simulink model "planta_inicial_tune"  (R2025b)
settings: Solver=VariableStepAuto  StartTime=0.0  StopTime=15  RelTol=1e-3
model workspace (MAT data in the model file):
  w = 0.5
values from neighbouring files (symbols this model uses):
  C1 = 1.2801    [Data_ControleLateral_atual.m]
  C2 = 23.99    [Data_ControleLateral_atual.m]
  C3 = 0.52    [Data_ControleLateral_atual.m]
undefined symbols (not defined in the file or in its folder): EV, GND, MTR, WHL
libraries: slpidlib x3, autolibutils x2, autolibmappedmotor x2, vehdynlibviscommon x1, autolibshared x1
settings Model: PacingRate=0.500000  Creator=Guilherme Porto  LastModifiedBy=Guilherme Porto

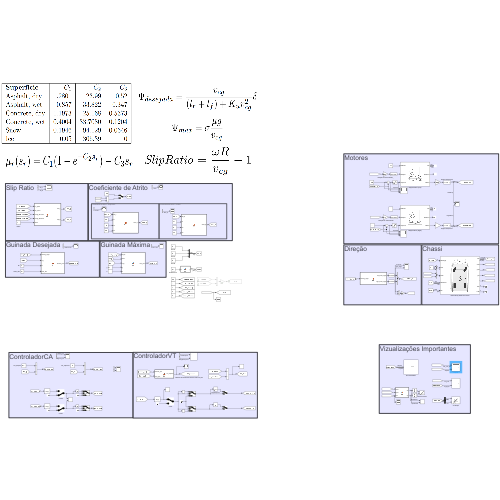
[thumbnail: Simulink's stored preview of the top-level diagram]
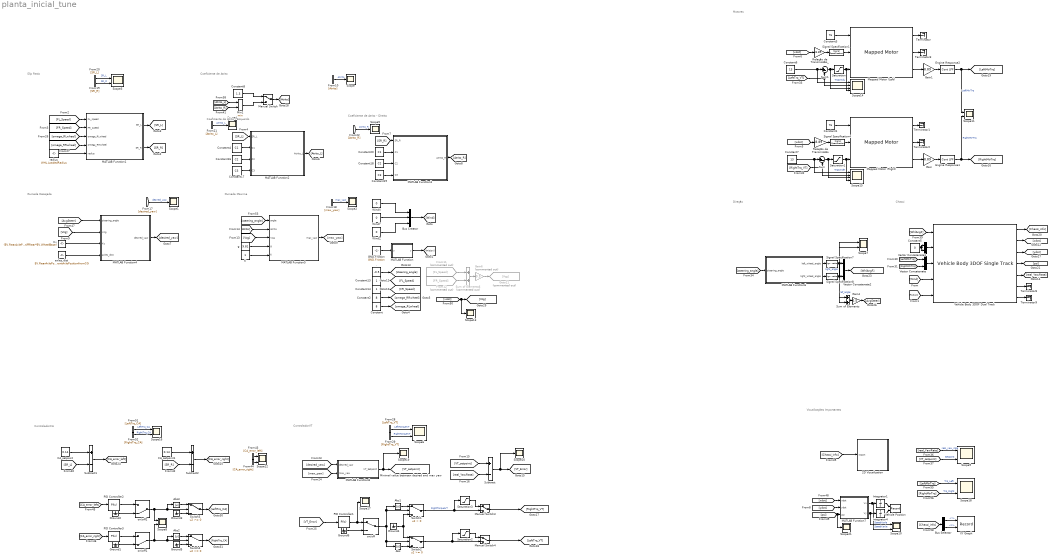
== system planta_inicial_tune ==
  note: Motores
  note: Direção
  note: Guinada Máxima
  note: Guinada Desejada
  note: Coeficiente de Atrito
  note: Coeficiente de Atrito - Esquerdo
  note: Slip Ratio
  note: Coeficiente de Atrito - Direito
  note: ControladorVT
  note: ControladorCA
  note: Chassi
  note: Vizualizações Importantes
  . : Constant  Value=-0.5
  2D Visualization : Subsystem
      mask Display: image("visualization.JPG");
  Abs{,1..3} (4 alike) : Abs  SaturateOnIntegerOverflow=off
  Bus Creator : BusCreator  Inputs=3
  Bus Selector : BusSelector  OutputSignals=InertFrm.Cg.Disp.Y,InertFrm.Cg.Disp.X
  CA_setpoint : Constant  Value=0.14
  CA_setpoint1 : Constant  Value=0.14
  Constant : Constant  Value=8
  Constant1 : Constant  Value=76
  Constant13 : Constant
  Constant14 : Constant
  Constant16 : Constant  Value=C2
  Constant17 : Constant  Value=C3
  Constant18 : Constant  Value=C2
  Constant19 : Constant  Value=C3
  Constant2 : Constant  Value=8
  Constant20 : Constant  Value=C1
  Constant3 : Constant  Value=76
  Constant4 : Constant  Value=C1
  Constant5 : Constant  Value=0
  Constant6 : Constant  Value=13
  Constant7 : Constant  Value=13
  Constant8 : Constant  Value=1.3
  Engine Response1 : autolibutils/Cont LPF  wc=40*2*pi  AbsoluteTolerance=auto  aMode=2
  Engine Response2 : autolibutils/Cont LPF  wc=40*2*pi  AbsoluteTolerance=auto  aMode=2
  From11 : From  Commented=on  GotoTag=FL_Speed
  From12 : From  Commented=on  GotoTag=FR_Speed
  GND.Friction : Constant  Value=GND.Friction
  Gain : Gain  Gain=8.89
  Gain1 : Gain  Gain=8.89
  Gain4 : Gain  Gain=0.5
  Gain6 : Gain  Commented=on  Gain=0.5
  Goto11 : Goto  Commented=on  GotoTag=Vcg
  Ground{1..6} (6 alike) : Ground
  Integrator1 : Integrator
  Integrator4 : Integrator
  Ku : Constant  Value=(EV.RearAxlePositionfromCG*EV.Mass)/(EV.CornerStiffFront *EV.WheelBase)-(EV.FrontAxlePositionfromCG*EV.Mass)/(EV.CornerStiffRear*EV.WheelBase)
  MATLAB Function : MATLAB Function  TreatAsAtomicUnit=on
  MATLAB Function1 : MATLAB Function  TreatAsAtomicUnit=on
  MATLAB Function2 : MATLAB Function  TreatAsAtomicUnit=on
  MATLAB Function3 : MATLAB Function  TreatAsAtomicUnit=on
  MATLAB Function4 : MATLAB Function  TreatAsAtomicUnit=on
  MATLAB Function5 : MATLAB Function  TreatAsAtomicUnit=on
  MATLAB Function6 : MATLAB Function  TreatAsAtomicUnit=on
  MATLAB Function7 : MATLAB Function  TreatAsAtomicUnit=on
  MATLAB Function8 : MATLAB Function  TreatAsAtomicUnit=on
  Manual Switch : ManualSwitch
  Manual Switch3 : ManualSwitch
  Manual Switch4 : ManualSwitch
  Mapped Motor (Left) : autolibmappedmotor/Mapped Motor  w_Tmax_bp_ext=[-800;-750;-375;0;375;750;800]  Tmax_w_V_ext=[0 0 0;0.07 0.07 0.07;0.08 0.08 0.08;0.09 0.09 0.09;0.08 0.08 0.08;0.07 0.07 0.07;0 0 0]  w_Tmin_bp_ext=[-800;-750;-375;0;375;750;800]  Tmin_w_V_ext=[0 0 0;-0.07 -0.07 -0.07;-0.08 -0.08 -0.08;-0.09 -0.09 -0.09;-0.08 -0.08 -0.08;-0.07 -0.07 -0.07;0 0 0]  port_config=Speed  param_by=Tabulated torque-speed envelope  w_t=MTR.Speed  T_t=MTR.Torque*MTR.Overpower  torque_max=.1  power_max=30  SpreadsheetTqLimitsFileName=MotorCalibrationImportData.xlsx  Tmax_w_V=[0.09 0.09 0.09;0.08 0.08 0.08;0.07 0.07 0.07;0 0 0]  w_Tmax_bp=[ 0 375 750 800 ]  V_Tmax_bp=[500 750 900]  Tmin_w_V=[-0.09 -0.09 -0.09;-0.08 -0.08 -0.08;-0.07 -0.07 -0.07;0 0 0]  w_Tmin_bp=[ 0 375 750 800 ]  V_Tmin_bp=[500 750 900]  Tc=0.05  param_loss=Single efficiency measurement  SpreadsheetLossFileName=MotorCalibrationImportData.xlsx  SpreadsheetEffFileName=MotorCalibrationImportData.xlsx  eff=100  w_eff=375  T_eff=0.08  Piron=0  Pbase=0  w_eff_bp=[-800 -400 0 400 800]  T_eff_bp=[0 0.03 0.06 0.09]  Temp_eff_bp=[233.15 293.15 373.15]  V_eff_bp=[500 700 900]  losses_table=[1.49 1.67 2.21 3.10; 0.42 0.69 1.14 2.03; 0.06 0.24 0.78 1.68; 0.42 0.69 1.14 2.03; 1.49 1.67 2.21 3.10]  losses_table_3d=cat(3,[1.49 1.67 2.21 3.10; 0.42 0.69 1.14 2.03; 0.06 0.24 0.78 1.68; 0.42 0.69 1.14 2.03; 1.49 1.67 2.21 3.10],[1.49 1.67 2.21 3.10; 0.42 0.69 1.14 2.03; 0.06 0.24 0.78 1.68; 0.42 0.69 1.14 2.03; 1.49 1.67 2.21 3.10],[1.49 1.67 2.21 3.10; 0.42 0.69 1.14 2.03; 0.06 0.24 0.78 1.68; 0.42 0.69 1.14 2.03; 1.49 1.67 2.21 3.10])  losses_table_4d=cat(4,cat(3,[1.5645 0.441 0.063 0.441 1.5645;1.7535 0.7245 0.252 0.7245 1.7535;2.3205 1.197 0.819 1.197 2.3205;3.255 2.1315 1.764 2.1315 3.255],[1.5645 0.441 0.063 0.441 1.5645;1.7535 0.7245 0.252 0.7245 1.7535;2.3205 1.197 0.819 1.197 2.3205;3.255 2.1315 1.764 2.1315 3.255],[1.5645 0.441 0.063 0.441 1.5645;1.7535 0.7245 0.252 0.7245 1.7535;2.3205 1.197 0.819 1.197 2.3205;3.255 2.1315 1.764 2.1315 3.255]),cat(3,[1.49 0.42 0.06 0.42 1.49;1.67 0.69 0.24 0.69 1.67;2.21 1.14 0.78 1.14 2.21;3.1 2.03 1.68 2.03 3.1],[1.49 0.42 0.06 0.42 1.49;1.67 0.69 0.24 0.69 1.67;2.21 1.14 0.78 1.14 2.21;3.1 2.03 1.68 2.03 3.1],[1.49 0.42 0.06 0.42 1.49;1.67 0.69 0.24 0.69 1.67;2.21 1.14 0.78 1.14 2.21;3.1 2.03 1.68 2.03 3.1]),cat(3,[1.5347 0.4326 0.0618 0.4326 1.5347;1.7201 0.7107 0.2472 0.7107 1.7201;2.2763 1.1742 0.8034 1.1742 2.2763;3.193 2.0909 1.7304 2.0909 3.193],[1.5347 0.4326 0.0618 0.4326 1.5347;1.7201 0.7107 0.2472 0.7107 1.7201;2.2763 1.1742 0.8034 1.1742 2.2763;3.193 2.0909 1.7304 2.0909 3.193],[1.5347 0.4326 0.0618 0.4326 1.5347;1.7201 0.7107 0.2472 0.7107 1.7201;2.2763 1.1742 0.8034 1.1742 2.2763;3.193 2.0909 1.7304 2.0909 3.193]))  efficiency_table=[95 95 95 95; 95 95 95 95; 95 95 95 95; 95 95 95 95; 95 95 95 95]  efficiency_table_3d=cat(3,[95 95 95 95; 95 95 95 95; 95 95 95 95; 95 95 95 95; 95 95 95 95],[95 95 95 95; 95 95 95 95; 95 95 95 95; 95 95 95 95; 95 95 95 95],[95 95 95 95; 95 95 95 95; 95 95 95 95; 95 95 95 95; 95 95 95 95])  efficiency_table_4d=cat(4,cat(3,90*ones(5,4)',90*ones(5,4)',90*ones(5,4)'),cat(3,95*ones(5,4)',95*ones(5,4)',95*ones(5,4)'),cat(3,92*ones(5,4)',92*ones(5,4)',92*ones(5,4)'))  J=5e-6  b=1e-5  omega_o=0  T_t_extended=[0 0.07 0.08 0.09 0.08 0.07 0]  w_t_extended=[-800 -750 -375 0 375 750 800]  KLossIron=0  KLossCopper=0  x_w_eff_vec=[-8000 -4000 0 4000 8000]  x_T_eff_vec=[-0.09 -0.06 -0.03 0 0.03 0.06 0.09]  x_tmp_eff_vec=[-0.09 -0.06 -0.03 0 0.03 0.06 0.09]  x_V_eff_vec=[500 700 900]  x_losses_mat=[3.1 2.21 1.67 1.49 1.67 2.21 3.1;2.03 1.14 0.69 0.42 0.69 1.14 2.03;1.68 0.78 0.24 0.06 0.24 0.78 1.68;2.03 1.14 0.69 0.42 0.69 1.14 2.03;3.1 2.21 1.67 1.49 1.67 2.21 3.1]  x_losses_mat_3d=[37.8947368421052 25.2631578947368 12.6315789473684 0 12 24 36;18.9473684210526 12.6315789473684 6.3157894736842 0 5.99999999999999 12 18;0 0 0 0 0 0 0;18 12 5.99999999999999 0 6.3157894736842 12.6315789473684 18.9473684210526;36 24 12 0 12.6315789473684 25.2631578947368 37.8947368421052]  x_losses_mat_4d="reshape([80;53.33;26.67;0;24;48;72;40;26.67;13.33;0;12;24;36;0;0;0;0;0;0;0;36;24;12;0;13.33;26.67;40;72;48;24;0;26.67;53.33;80;80;53.33;26.67;0;24;48;72;40;26.67;13.33;0;12;24;36;0;0;0;0;0;0;0;36;24;12;0;13.33;26.67;40;72;48;24;0;26.67;53.33;80;80;53.33;26.67;0;24;48;72;40;26.67;13.33;0;12;24;36;0;0;0;0;0;0;0;36;24;12;0;13.33;26.67;40;72;48;24;0;26.67;53.33;80;37.89;25.26;12.63;0;12;24;36;18.95;12.63;6.32;0;6;12;18;0;0;0;0;0;0;0;18;12;6;0;6.32;12.63;18.95;36;24;12;0;12.63;25.26;37.89;37.89;25.26;12.63;0;12;24;36;18.95;12.63;6.32;0;6;12;18;0;0;0;0;0;0;0;18;12;6;0;6.32;12.63;18.95;36;24;12;0;12.63;25.26;37.89;37.89;25.26;12.63;0;12;24;36;18.95;12.63;6.32;0;6;12;18;0;0;0;0;0;0;0;18;12;6;0;6.32;12.63;18.95;36;24;12;0;12.63;25.26;37.89;62.61;41.74;20.87;0;19.2;38.4;57.6;31.3;20.87;10.43;0;9.6;19.2;28.8;0;0;0;0;0;0;0;28.8;19.2;9.6;0;10.43;20.87;31.3;57.6;38.4;19.2;0;20.87;41.74;62.61;62.61;41.74;20.87;0;19.2;38.4;57.6;31.3;20.87;10.43;0;9.6;19.2;28.8;0;0;0;0;0;0;0;28.8;19.2;9.6;0;10.43;20.87;31.3;57.6;38.4;19.2;0;20.87;41.74;62.61;62.61;41.74;20.87;0;19.2;38.4;57.6;31.3;20.87;10.43;0;9.6;19.2;28.8;0;0;0;0;0;0;0;28.8;19.2;9.6;0;10.43;20.87;31.3;57.6;38.4;19.2;0;20.87;41.74;62.61], [7  5  3  3])"  CalLossMapData={}  CalLossWithTempMapData={}  aMode=1  RefBlkName='autolibmappedmotor/Mapped Motor'
      settings: LibrarySourceBlock=autolibemachines/Mapped Motor
  Mapped Motor (Right) : autolibmappedmotor/Mapped Motor  w_Tmax_bp_ext=[-800;-750;-375;0;375;750;800]  Tmax_w_V_ext=[0 0 0;0.07 0.07 0.07;0.08 0.08 0.08;0.09 0.09 0.09;0.08 0.08 0.08;0.07 0.07 0.07;0 0 0]  w_Tmin_bp_ext=[-800;-750;-375;0;375;750;800]  Tmin_w_V_ext=[0 0 0;-0.07 -0.07 -0.07;-0.08 -0.08 -0.08;-0.09 -0.09 -0.09;-0.08 -0.08 -0.08;-0.07 -0.07 -0.07;0 0 0]  port_config=Speed  param_by=Tabulated torque-speed envelope  w_t=MTR.Speed  T_t=MTR.Torque*MTR.Overpower  torque_max=.1  power_max=30  SpreadsheetTqLimitsFileName=MotorCalibrationImportData.xlsx  Tmax_w_V=[0.09 0.09 0.09;0.08 0.08 0.08;0.07 0.07 0.07;0 0 0]  w_Tmax_bp=[ 0 375 750 800 ]  V_Tmax_bp=[500 750 900]  Tmin_w_V=[-0.09 -0.09 -0.09;-0.08 -0.08 -0.08;-0.07 -0.07 -0.07;0 0 0]  w_Tmin_bp=[ 0 375 750 800 ]  V_Tmin_bp=[500 750 900]  Tc=0.05  param_loss=Single efficiency measurement  SpreadsheetLossFileName=MotorCalibrationImportData.xlsx  SpreadsheetEffFileName=MotorCalibrationImportData.xlsx  eff=100  w_eff=375  T_eff=0.08  Piron=0  Pbase=0  w_eff_bp=[-800 -400 0 400 800]  T_eff_bp=[0 0.03 0.06 0.09]  Temp_eff_bp=[233.15 293.15 373.15]  V_eff_bp=[500 700 900]  losses_table=[1.49 1.67 2.21 3.10; 0.42 0.69 1.14 2.03; 0.06 0.24 0.78 1.68; 0.42 0.69 1.14 2.03; 1.49 1.67 2.21 3.10]  losses_table_3d=cat(3,[1.49 1.67 2.21 3.10; 0.42 0.69 1.14 2.03; 0.06 0.24 0.78 1.68; 0.42 0.69 1.14 2.03; 1.49 1.67 2.21 3.10],[1.49 1.67 2.21 3.10; 0.42 0.69 1.14 2.03; 0.06 0.24 0.78 1.68; 0.42 0.69 1.14 2.03; 1.49 1.67 2.21 3.10],[1.49 1.67 2.21 3.10; 0.42 0.69 1.14 2.03; 0.06 0.24 0.78 1.68; 0.42 0.69 1.14 2.03; 1.49 1.67 2.21 3.10])  losses_table_4d=cat(4,cat(3,[1.5645 0.441 0.063 0.441 1.5645;1.7535 0.7245 0.252 0.7245 1.7535;2.3205 1.197 0.819 1.197 2.3205;3.255 2.1315 1.764 2.1315 3.255],[1.5645 0.441 0.063 0.441 1.5645;1.7535 0.7245 0.252 0.7245 1.7535;2.3205 1.197 0.819 1.197 2.3205;3.255 2.1315 1.764 2.1315 3.255],[1.5645 0.441 0.063 0.441 1.5645;1.7535 0.7245 0.252 0.7245 1.7535;2.3205 1.197 0.819 1.197 2.3205;3.255 2.1315 1.764 2.1315 3.255]),cat(3,[1.49 0.42 0.06 0.42 1.49;1.67 0.69 0.24 0.69 1.67;2.21 1.14 0.78 1.14 2.21;3.1 2.03 1.68 2.03 3.1],[1.49 0.42 0.06 0.42 1.49;1.67 0.69 0.24 0.69 1.67;2.21 1.14 0.78 1.14 2.21;3.1 2.03 1.68 2.03 3.1],[1.49 0.42 0.06 0.42 1.49;1.67 0.69 0.24 0.69 1.67;2.21 1.14 0.78 1.14 2.21;3.1 2.03 1.68 2.03 3.1]),cat(3,[1.5347 0.4326 0.0618 0.4326 1.5347;1.7201 0.7107 0.2472 0.7107 1.7201;2.2763 1.1742 0.8034 1.1742 2.2763;3.193 2.0909 1.7304 2.0909 3.193],[1.5347 0.4326 0.0618 0.4326 1.5347;1.7201 0.7107 0.2472 0.7107 1.7201;2.2763 1.1742 0.8034 1.1742 2.2763;3.193 2.0909 1.7304 2.0909 3.193],[1.5347 0.4326 0.0618 0.4326 1.5347;1.7201 0.7107 0.2472 0.7107 1.7201;2.2763 1.1742 0.8034 1.1742 2.2763;3.193 2.0909 1.7304 2.0909 3.193]))  efficiency_table=[95 95 95 95; 95 95 95 95; 95 95 95 95; 95 95 95 95; 95 95 95 95]  efficiency_table_3d=cat(3,[95 95 95 95; 95 95 95 95; 95 95 95 95; 95 95 95 95; 95 95 95 95],[95 95 95 95; 95 95 95 95; 95 95 95 95; 95 95 95 95; 95 95 95 95],[95 95 95 95; 95 95 95 95; 95 95 95 95; 95 95 95 95; 95 95 95 95])  efficiency_table_4d=cat(4,cat(3,90*ones(5,4)',90*ones(5,4)',90*ones(5,4)'),cat(3,95*ones(5,4)',95*ones(5,4)',95*ones(5,4)'),cat(3,92*ones(5,4)',92*ones(5,4)',92*ones(5,4)'))  J=5e-6  b=1e-5  omega_o=0  T_t_extended=[0 0.07 0.08 0.09 0.08 0.07 0]  w_t_extended=[-800 -750 -375 0 375 750 800]  KLossIron=0  KLossCopper=0  x_w_eff_vec=[-8000 -4000 0 4000 8000]  x_T_eff_vec=[-0.09 -0.06 -0.03 0 0.03 0.06 0.09]  x_tmp_eff_vec=[-0.09 -0.06 -0.03 0 0.03 0.06 0.09]  x_V_eff_vec=[500 700 900]  x_losses_mat=[3.1 2.21 1.67 1.49 1.67 2.21 3.1;2.03 1.14 0.69 0.42 0.69 1.14 2.03;1.68 0.78 0.24 0.06 0.24 0.78 1.68;2.03 1.14 0.69 0.42 0.69 1.14 2.03;3.1 2.21 1.67 1.49 1.67 2.21 3.1]  x_losses_mat_3d=[37.8947368421052 25.2631578947368 12.6315789473684 0 12 24 36;18.9473684210526 12.6315789473684 6.3157894736842 0 5.99999999999999 12 18;0 0 0 0 0 0 0;18 12 5.99999999999999 0 6.3157894736842 12.6315789473684 18.9473684210526;36 24 12 0 12.6315789473684 25.2631578947368 37.8947368421052]  x_losses_mat_4d="reshape([80;53.33;26.67;0;24;48;72;40;26.67;13.33;0;12;24;36;0;0;0;0;0;0;0;36;24;12;0;13.33;26.67;40;72;48;24;0;26.67;53.33;80;80;53.33;26.67;0;24;48;72;40;26.67;13.33;0;12;24;36;0;0;0;0;0;0;0;36;24;12;0;13.33;26.67;40;72;48;24;0;26.67;53.33;80;80;53.33;26.67;0;24;48;72;40;26.67;13.33;0;12;24;36;0;0;0;0;0;0;0;36;24;12;0;13.33;26.67;40;72;48;24;0;26.67;53.33;80;37.89;25.26;12.63;0;12;24;36;18.95;12.63;6.32;0;6;12;18;0;0;0;0;0;0;0;18;12;6;0;6.32;12.63;18.95;36;24;12;0;12.63;25.26;37.89;37.89;25.26;12.63;0;12;24;36;18.95;12.63;6.32;0;6;12;18;0;0;0;0;0;0;0;18;12;6;0;6.32;12.63;18.95;36;24;12;0;12.63;25.26;37.89;37.89;25.26;12.63;0;12;24;36;18.95;12.63;6.32;0;6;12;18;0;0;0;0;0;0;0;18;12;6;0;6.32;12.63;18.95;36;24;12;0;12.63;25.26;37.89;62.61;41.74;20.87;0;19.2;38.4;57.6;31.3;20.87;10.43;0;9.6;19.2;28.8;0;0;0;0;0;0;0;28.8;19.2;9.6;0;10.43;20.87;31.3;57.6;38.4;19.2;0;20.87;41.74;62.61;62.61;41.74;20.87;0;19.2;38.4;57.6;31.3;20.87;10.43;0;9.6;19.2;28.8;0;0;0;0;0;0;0;28.8;19.2;9.6;0;10.43;20.87;31.3;57.6;38.4;19.2;0;20.87;41.74;62.61;62.61;41.74;20.87;0;19.2;38.4;57.6;31.3;20.87;10.43;0;9.6;19.2;28.8;0;0;0;0;0;0;0;28.8;19.2;9.6;0;10.43;20.87;31.3;57.6;38.4;19.2;0;20.87;41.74;62.61], [7  5  3  3])"  CalLossMapData={'BaseCageProjectFileName','';'BaseMbcProjectFileName','';'TaskName','Calibrate Motor Loss Map';'ChildTasks',{{'DataName','';'TaskName','Import Loss Data'},{'TaskName','Generate Response Models'},{'TaskName','Generate Calibration'},{'TaskName','Update Block Parameters'}}}  CalLossWithTempMapData={}  aMode=1  RefBlkName='autolibmappedmotor/Mapped Motor'
      settings: LibrarySourceBlock=autolibemachines/Mapped Motor
  Min1 : MinMax  Inputs=2
  PID Controller1 : slpidlib/PID Controller  Controller=PI  Form=Parallel  TimeDomain=Continuous-time  UseExternalTs=off  SampleTime=-1  IntegratorMethod=Forward Euler  FilterMethod=Forward Euler  ControllerParametersSource=internal  P=1188  I=86  UseKiTs=off  D=-1.04450033164761  UseExternalDerivativeSource=off  N=21.9051072982779  UseFilter=on  TunerSelectOption=Transfer Function Based (PID Tuner App)  InitialConditionSource=internal  InitialConditionForIntegrator=0  InitialConditionForFilter=0  DifferentiatorICPrevScaledInput=0  ExternalReset=none  TrackingMode=off  Kt=1  LimitOutput=off  SatLimitsSource=internal  UpperSaturationLimit=inf  LowerSaturationLimit=-inf  LinearizeAsGain=on  AntiWindupMode=none  Kb=1  LimitIntegrator=off  UpperIntegratorSaturationLimit=inf  LowerIntegratorSaturationLimit=-inf  POutMin=[]  POutMax=[]  IOutMin=[]  IOutMax=[]  DOutMin=[]  DOutMax=[]  NOutMin=[]  NOutMax=[]  SumOutMin=[]  SumOutMax=[]  SaturationOutMin=[]  SaturationOutMax=[]  PParamMin=[]  PParamMax=[]  IParamMin=[]  IParamMax=[]  DParamMin=[]  DParamMax=[]  NParamMin=[]  NParamMax=[]  KbParamMin=[]  KbParamMax=[]  KtParamMin=[]  KtParamMax=[]  KbOutMin=[]  KbOutMax=[]  KtOutMin=[]  KtOutMax=[]  IntegratorOutMin=[]  IntegratorOutMax=[]  FilterOutMin=[]  FilterOutMax=[]  SumI1OutMin=[]  SumI1OutMax=[]  SumI2OutMin=[]  SumI2OutMax=[]  SumI3OutMin=[]  SumI3OutMax=[]  SumI4OutMin=[]  SumI4OutMax=[]  SumDOutMin=[]  SumDOutMax=[]  DifferentiatorOutMin=[]  DifferentiatorOutMax=[]  FilterDiffOutCoefMin=[]  FilterDiffOutCoefMax=[]  ReciprocalOutMin=[]  ReciprocalOutMax=[]  SumDenOutMin=[]  SumDenOutMax=[]  SumNumOutMin=[]  SumNumOutMax=[]  DivideOutMin=[]  DivideOutMax=[]  UdiffTsProdOutMin=[]  UdiffTsProdOutMax=[]  NTsProdOutMin=[]  NTsProdOutMax=[]  UintegralTsProdOutMin=[]  UintegralTsProdOutMax=[]  UngainTsProdOutMin=[]  UngainTsProdOutMax=[]  ClampingZeroOutDataTypeStr=Inherit: Inherit via back propagation  ClampingZeroOutMin=[]  ClampingZeroOutMax=[]  FilterDenConstantOutDataTypeStr=Inherit: Inherit via back propagation  FilterDenConstantOutMin=[]  FilterDenConstantOutMax=[]  PCopyOutDataTypeStr=Inherit: Inherit via back propagation  PCopyOutMin=[]  PCopyOutMax=[]  NCopyOutDataTypeStr=Inherit: Inherit via back propagation  NCopyOutMin=[]  NCopyOutMax=[]  IntegratorContinuousStateAttributes=''  IntegratorStateMustResolveToSignalObject=off  IntegratorRTWStateStorageClass=Auto  FilterContinuousStateAttributes=''  FilterStateMustResolveToSignalObject=off  FilterRTWStateStorageClass=Auto  ParallelPVariant=InternalParameters  IdealPVariant=Disabled  IVariant=InternalParameters  DVariant=Disabled  IntegratorVariant=Continuous  SatVariant=Disabled  AWVariant=Passthrough  PCopyVariant=Disabled  TRVariant=Disabled  FdbkBlocksVariant=Forward  IdealPFdbkVariant=Disabled  SatFdbkVariant=Disabled  DerivativeFilterVariant=Disabled  NVariant=Disabled  NCopyVariant=Disabled_SignalSpec  FilterICVariant=Disabled  IntegratorICVariant=InternalICs  ExternalResetVariant=Disabled  TRSumVariant=Passthrough  SumFdbkVariant=Disabled  SumVariant=Sum_PI  TsampFilterVariant=InternalTs  TsampNgainVariant=Passthrough  TsampIntegralVariant=Disabled_SignalSpec  ExternalSaturationOutDataTypeStr=Inherit: Same as second input  DerivativeSourceVariant=Disabled  PreIntVariant=InternalPreInt
  PID Controller2 : slpidlib/PID Controller  Controller=PI  Form=Parallel  TimeDomain=Continuous-time  UseExternalTs=off  SampleTime=-1  IntegratorMethod=Forward Euler  FilterMethod=Forward Euler  ControllerParametersSource=internal  P=1000  I=100  UseKiTs=off  D=-1.04450033164761  UseExternalDerivativeSource=off  N=21.9051072982779  UseFilter=on  TunerSelectOption=Transfer Function Based (PID Tuner App)  InitialConditionSource=internal  InitialConditionForIntegrator=0  InitialConditionForFilter=0  DifferentiatorICPrevScaledInput=0  ExternalReset=none  TrackingMode=off  Kt=1  LimitOutput=off  SatLimitsSource=internal  UpperSaturationLimit=inf  LowerSaturationLimit=-inf  LinearizeAsGain=on  AntiWindupMode=none  Kb=1  LimitIntegrator=off  UpperIntegratorSaturationLimit=inf  LowerIntegratorSaturationLimit=-inf  POutMin=[]  POutMax=[]  IOutMin=[]  IOutMax=[]  DOutMin=[]  DOutMax=[]  NOutMin=[]  NOutMax=[]  SumOutMin=[]  SumOutMax=[]  SaturationOutMin=[]  SaturationOutMax=[]  PParamMin=[]  PParamMax=[]  IParamMin=[]  IParamMax=[]  DParamMin=[]  DParamMax=[]  NParamMin=[]  NParamMax=[]  KbParamMin=[]  KbParamMax=[]  KtParamMin=[]  KtParamMax=[]  KbOutMin=[]  KbOutMax=[]  KtOutMin=[]  KtOutMax=[]  IntegratorOutMin=[]  IntegratorOutMax=[]  FilterOutMin=[]  FilterOutMax=[]  SumI1OutMin=[]  SumI1OutMax=[]  SumI2OutMin=[]  SumI2OutMax=[]  SumI3OutMin=[]  SumI3OutMax=[]  SumI4OutMin=[]  SumI4OutMax=[]  SumDOutMin=[]  SumDOutMax=[]  DifferentiatorOutMin=[]  DifferentiatorOutMax=[]  FilterDiffOutCoefMin=[]  FilterDiffOutCoefMax=[]  ReciprocalOutMin=[]  ReciprocalOutMax=[]  SumDenOutMin=[]  SumDenOutMax=[]  SumNumOutMin=[]  SumNumOutMax=[]  DivideOutMin=[]  DivideOutMax=[]  UdiffTsProdOutMin=[]  UdiffTsProdOutMax=[]  NTsProdOutMin=[]  NTsProdOutMax=[]  UintegralTsProdOutMin=[]  UintegralTsProdOutMax=[]  UngainTsProdOutMin=[]  UngainTsProdOutMax=[]  ClampingZeroOutDataTypeStr=Inherit: Inherit via back propagation  ClampingZeroOutMin=[]  ClampingZeroOutMax=[]  FilterDenConstantOutDataTypeStr=Inherit: Inherit via back propagation  FilterDenConstantOutMin=[]  FilterDenConstantOutMax=[]  PCopyOutDataTypeStr=Inherit: Inherit via back propagation  PCopyOutMin=[]  PCopyOutMax=[]  NCopyOutDataTypeStr=Inherit: Inherit via back propagation  NCopyOutMin=[]  NCopyOutMax=[]  IntegratorContinuousStateAttributes=''  IntegratorStateMustResolveToSignalObject=off  IntegratorRTWStateStorageClass=Auto  FilterContinuousStateAttributes=''  FilterStateMustResolveToSignalObject=off  FilterRTWStateStorageClass=Auto  ParallelPVariant=InternalParameters  IdealPVariant=Disabled  IVariant=InternalParameters  DVariant=Disabled  IntegratorVariant=Continuous  SatVariant=Disabled  AWVariant=Passthrough  PCopyVariant=Disabled  TRVariant=Disabled  FdbkBlocksVariant=Forward  IdealPFdbkVariant=Disabled  SatFdbkVariant=Disabled  DerivativeFilterVariant=Disabled  NVariant=Disabled  NCopyVariant=Disabled_SignalSpec  FilterICVariant=Disabled  IntegratorICVariant=InternalICs  ExternalResetVariant=Disabled  TRSumVariant=Passthrough  SumFdbkVariant=Disabled  SumVariant=Sum_PI  TsampFilterVariant=InternalTs  TsampNgainVariant=Passthrough  TsampIntegralVariant=Disabled_SignalSpec  ExternalSaturationOutDataTypeStr=Inherit: Same as second input  DerivativeSourceVariant=Disabled  PreIntVariant=InternalPreInt
  PID Controller3 : slpidlib/PID Controller  Controller=PI  Form=Parallel  TimeDomain=Continuous-time  UseExternalTs=off  SampleTime=-1  IntegratorMethod=Forward Euler  FilterMethod=Forward Euler  ControllerParametersSource=internal  P=1000  I=100  UseKiTs=off  D=-1.04450033164761  UseExternalDerivativeSource=off  N=21.9051072982779  UseFilter=on  TunerSelectOption=Transfer Function Based (PID Tuner App)  InitialConditionSource=internal  InitialConditionForIntegrator=0  InitialConditionForFilter=0  DifferentiatorICPrevScaledInput=0  ExternalReset=none  TrackingMode=off  Kt=1  LimitOutput=off  SatLimitsSource=internal  UpperSaturationLimit=inf  LowerSaturationLimit=-inf  LinearizeAsGain=on  AntiWindupMode=none  Kb=1  LimitIntegrator=off  UpperIntegratorSaturationLimit=inf  LowerIntegratorSaturationLimit=-inf  POutMin=[]  POutMax=[]  IOutMin=[]  IOutMax=[]  DOutMin=[]  DOutMax=[]  NOutMin=[]  NOutMax=[]  SumOutMin=[]  SumOutMax=[]  SaturationOutMin=[]  SaturationOutMax=[]  PParamMin=[]  PParamMax=[]  IParamMin=[]  IParamMax=[]  DParamMin=[]  DParamMax=[]  NParamMin=[]  NParamMax=[]  KbParamMin=[]  KbParamMax=[]  KtParamMin=[]  KtParamMax=[]  KbOutMin=[]  KbOutMax=[]  KtOutMin=[]  KtOutMax=[]  IntegratorOutMin=[]  IntegratorOutMax=[]  FilterOutMin=[]  FilterOutMax=[]  SumI1OutMin=[]  SumI1OutMax=[]  SumI2OutMin=[]  SumI2OutMax=[]  SumI3OutMin=[]  SumI3OutMax=[]  SumI4OutMin=[]  SumI4OutMax=[]  SumDOutMin=[]  SumDOutMax=[]  DifferentiatorOutMin=[]  DifferentiatorOutMax=[]  FilterDiffOutCoefMin=[]  FilterDiffOutCoefMax=[]  ReciprocalOutMin=[]  ReciprocalOutMax=[]  SumDenOutMin=[]  SumDenOutMax=[]  SumNumOutMin=[]  SumNumOutMax=[]  DivideOutMin=[]  DivideOutMax=[]  UdiffTsProdOutMin=[]  UdiffTsProdOutMax=[]  NTsProdOutMin=[]  NTsProdOutMax=[]  UintegralTsProdOutMin=[]  UintegralTsProdOutMax=[]  UngainTsProdOutMin=[]  UngainTsProdOutMax=[]  ClampingZeroOutDataTypeStr=Inherit: Inherit via back propagation  ClampingZeroOutMin=[]  ClampingZeroOutMax=[]  FilterDenConstantOutDataTypeStr=Inherit: Inherit via back propagation  FilterDenConstantOutMin=[]  FilterDenConstantOutMax=[]  PCopyOutDataTypeStr=Inherit: Inherit via back propagation  PCopyOutMin=[]  PCopyOutMax=[]  NCopyOutDataTypeStr=Inherit: Inherit via back propagation  NCopyOutMin=[]  NCopyOutMax=[]  IntegratorContinuousStateAttributes=''  IntegratorStateMustResolveToSignalObject=off  IntegratorRTWStateStorageClass=Auto  FilterContinuousStateAttributes=''  FilterStateMustResolveToSignalObject=off  FilterRTWStateStorageClass=Auto  ParallelPVariant=InternalParameters  IdealPVariant=Disabled  IVariant=InternalParameters  DVariant=Disabled  IntegratorVariant=Continuous  SatVariant=Disabled  AWVariant=Passthrough  PCopyVariant=Disabled  TRVariant=Disabled  FdbkBlocksVariant=Forward  IdealPFdbkVariant=Disabled  SatFdbkVariant=Disabled  DerivativeFilterVariant=Disabled  NVariant=Disabled  NCopyVariant=Disabled_SignalSpec  FilterICVariant=Disabled  IntegratorICVariant=InternalICs  ExternalResetVariant=Disabled  TRSumVariant=Passthrough  SumFdbkVariant=Disabled  SumVariant=Sum_PI  TsampFilterVariant=InternalTs  TsampNgainVariant=Passthrough  TsampIntegralVariant=Disabled_SignalSpec  ExternalSaturationOutDataTypeStr=Inherit: Same as second input  DerivativeSourceVariant=Disabled  PreIntVariant=InternalPreInt
  Relação de Transmissão : Gain  Gain=8.89
  Relação de Transmissão_ : Gain  Gain=8.89
  Saturation : Saturate  UpperLimit=45  LowerLimit=0
  Saturation1 : Saturate  UpperLimit=45  LowerLimit=0
  Saturation2 : Saturate  UpperLimit=11.7  LowerLimit=0
  Saturation3 : Saturate  UpperLimit=11.7  LowerLimit=0
  Scope{,1..2,4..5,13,17,19..21} (10 alike) : Scope
      Scope settings: ActiveDisplayYMinimum=0.30000000000000004  ActiveDisplayYMaximum=2.3
      Scope1 settings: ActiveDisplayYMinimum=0.76570776060353807  ActiveDisplayYMaximum=0.77363725190068056
      Scope13 settings: ActiveDisplayYMinimum=8.0450508328128176  ActiveDisplayYMaximum=10.019162352613328  DataLoggingVariableName=ScopeData13
      Scope17 settings: ActiveDisplayYMinimum=-2557.0099306998736  ActiveDisplayYMaximum=16.194536763193582  DataLoggingVariableName=ScopeData17
      Scope19 settings: ActiveDisplayYMinimum=-0.9176139828630353  ActiveDisplayYMaximum=-0.7574354136214948  DataLoggingVariableName=ScopeData19
      Scope2 settings: ActiveDisplayYMinimum=-1.5597915671939708  ActiveDisplayYMaximum=-1.2875145681353783  DataLoggingVariableName=ScopeData2
      Scope20 settings: DataLoggingVariableName=ScopeData20
      Scope21 settings: ActiveDisplayYMinimum=-1.1372487774874092  ActiveDisplayYMaximum=13.235238997386684  DataLoggingVariableName=ScopeData21
      Scope4 settings: ActiveDisplayYMinimum=0.75658729494332844  ActiveDisplayYMaximum=0.763972516800221  DataLoggingVariableName=ScopeData4
      Scope5 settings: ActiveDisplayYMinimum=0.651092857094046  ActiveDisplayYMaximum=0.882617857094046  DataLoggingVariableName=ScopeData5
  Scope{3,6..12,16,18} (10 alike) : Scope  NumInputPorts=2
      Scope10 settings: ActiveDisplayYMinimum=-16.081446238125832  ActiveDisplayYMaximum=28.863351857100209  DataLoggingVariableName=ScopeData10
      Scope11 settings: ActiveDisplayYMinimum=-80.862104288579161  ActiveDisplayYMaximum=219.46505782963624  DataLoggingVariableName=ScopeData11
      Scope12 settings: ActiveDisplayYMinimum=-0.96  ActiveDisplayYMaximum=-0.76  DataLoggingVariableName=ScopeData12
      Scope16 settings: ActiveDisplayYMinimum=-0.60664795279111228  ActiveDisplayYMaximum=0.96040438014580543  DataLoggingVariableName=ScopeData16
      Scope18 settings: ActiveDisplayYMinimum=-14.446250628959627  ActiveDisplayYMaximum=130.01625566063666  DataLoggingVariableName=ScopeData18
      Scope3 settings: ActiveDisplayYMinimum=0.85095205185300393  ActiveDisplayYMaximum=1.1930199234762668  DataLoggingVariableName=ScopeData3
      Scope6 settings: ActiveDisplayYMinimum=-112.69949637878479  ActiveDisplayYMaximum=1014.2954674090633  DataLoggingVariableName=ScopeData7
      Scope7 settings: ActiveDisplayYMinimum=-0.156063369582835  ActiveDisplayYMaximum=-0.13207559850072498  DataLoggingVariableName=ScopeData6
      Scope8 settings: ActiveDisplayYMinimum=-2311.2500000000018  ActiveDisplayYMaximum=-698.74999999999977  DataLoggingVariableName=ScopeData8
      Scope9 settings: ActiveDisplayYMinimum=-1.0142956416812414  ActiveDisplayYMaximum=0.11269951574236013  DataLoggingVariableName=ScopeData9
  Scope14 : Scope  NumInputPorts=4
      settings: ActiveDisplayYMinimum=-56.821757837281808  ActiveDisplayYMaximum=137.46004940329951  DataLoggingVariableName=ScopeData14
  Scope15 : Scope  NumInputPorts=4
      settings: ActiveDisplayYMinimum=-5.7358374466277464  ActiveDisplayYMaximum=20.733700238505691  DataLoggingVariableName=ScopeData15
  Signal Specification1 : SignalSpecification  Unit=rad/s
  Signal Specification4 : SignalSpecification  Unit=rad/s
  Signal Specification7 : SignalSpecification  Unit=rad
  Signal Specification8 : SignalSpecification  Unit=rad
  Subtract : Sum  Inputs=+-
  Subtract1 : Sum  Inputs=+-
  Subtract2 : Sum  Inputs=+-
  Sum : Sum  Inputs=|+-
  Sum of Elements : Sum
  Sum of Elements6 : Sum  Commented=on
  Sum1 : Sum  Inputs=|+-
  Switch1 : Switch  Criteria=u2 > Threshold  SaturateOnIntegerOverflow=off  InputSameDT=off
  Switch2 : Switch  SaturateOnIntegerOverflow=off  InputSameDT=off
  Switch3 : Switch  SaturateOnIntegerOverflow=off  InputSameDT=off
  Switch4 : Switch  SaturateOnIntegerOverflow=off  InputSameDT=off
  Terminator{,1..3,8..9} (6 alike) : Terminator
  Vector Concatenate : Concatenate
  Vector Concatenate1 : Concatenate
  Vector Concatenate2 : Concatenate
  Vehicle Body 3DOF Dual Track : autolibshared/Vehicle Body 3DOF Single Track  trackMode=Dual  inputMode=External longitudinal forces  frontSteerMode=on  rearSteerMode=off  windMode=on  muMode=on  extFMode=off  extMMode=off  htchFMode=off  htchMMode=off  extXo=off  extpsio=off  extxdoto=off  extro=off  extYo=off  extTamb=off  extydoto=off  aMode=2  NF=EV.NumberOfWheelsPerAxle  NR=EV.NumberOfWheelsPerAxle  m=EV.Mass  a=EV.FrontAxlePositionfromCG  b=EV.RearAxlePositionfromCG  h=EV.HeightCG  dh=1  hh=0.2  X_o=EV.InitialLongPosition  xdot_o=9.7  CalphaMode=off  sigmaMode=on  d=0  hl=0  w=EV.TrackWidth.*[1 1]  Cy_f=20000  Cy_r=20000  sigma_f=.1  sigma_r=.1  alpha_f_brk=[-0.785, -0.628, -0.471, -0.314, -0.157, 0.000, 0.157, 0.314, 0.471, 0.628, 0.785]  Cy_f_data=[2000, 3000, 4000, 5500, 7000, 9000, 7000, 5500, 4000, 3000, 2000]  alpha_r_brk=[-0.785, -0.628, -0.471, -0.314, -0.157, 0.000, 0.157, 0.314, 0.471, 0.628, 0.785]  Cy_r_data=[2000, 3000, 4000, 5500, 7000, 9000, 7000, 5500, 4000, 3000, 2000]  Y_o=EV.InitialLatPosition  ydot_o=EV.InitialLatVel  Izz=EV.YawMomentInertia  psi_o=EV.InitialYawAngle  r_o=EV.InitialYawRate  Af=EV.FrontalArea  Cd=EV.LongDragCoeff  Cl=.1  Cpm=.1  beta_w=[0:0.01:0.3]  Cs=[0:0.03:0.9]  Cym=[0:0.01:0.3]  Pabs=101325  Tair=273  g=9.81  mu=1  xdot_tol=1  Fznom=5000  Fxtire_sat=7e4  Fytire_sat=7e4  longOff=0  latOff=0  vertOff=.0112  wrapAng=off
      settings: LibrarySourceBlock=vehdynlibeom/Vehicle Body 3DOF Dual Track
  Vehicle Position : Record  NumPorts=2.0  FileSettingsInternal="{\"entries\":[{\"content\":{\"excelSettings\":{\"content\":{},\"type\":\"Streamout.ExcelSettings\"},\"parquetSettings\":{\"content\":{},\"type\":\"Streamout.ParquetSettings\"}},\"type\":\"Streamout.FileSettingStorage\",\"uuid\":\"\"}],\"packageUris\":[\"http:\\/\\/schema.mathworks.com\\/mf0\\/streamout_blocks\\/R2020a\"],\"version\":\"1.0\"}"  FrameSettings=[0, 0]  Layout=[1 1]  SignalsInternal="{\"entries\":[{\"content\":{\"signals\":[{\"content\":{\"blockPath\":[],\"dimensions\":[1],\"domain\":\"\",\"lineColor\":\"#a2142f\",\"plots\":[ 1 ],\"port\":1,\"sid\":[\"\"],\"signalID\":1,\"signalName\":\"Integrator1\"},\"type\":\"RecordBlkView.Signal\",\"uuid\":\"\"},{\"content\":{\"blockPath\":[],\"dimensions\":[1],\"domain\":\"\",\"lineColor\":\"#139fff\",\"plots\":[ 1 ],\"port\":2,\"sid\":[\"\"],\"signalID\":2,\"signalName\":\"Integrator4\"},\"type\":\"RecordBlkView.Signal\",\"uuid\":\"\"}]},\"type\":\"RecordBlkView.InputSignals\",\"uuid\":\"\"}],\"packageUris\":[\"http:\\/\\/schema.mathworks.com\\/mf0\\/streamout_blocks\\/R2020a\"],\"version\":\"1.0\"}"  VisualizationBindings="{\"xyplotplugin\":{\"info\":[{\"series\":[{\"bindingParametersList\":[{\"parameter\":\"X-Axis\",\"signalID\":1,\"signalName\":\"Integrator1\"},{\"parameter\":\"Y-Axis\",\"signalID\":2,\"signalName\":\"Integrator4\"}],\"seriesID\":0}],\"subplotID\":1}]}}"  CompatibilityTag=XY
  WindX : Constant  Value=0
  WindY : Constant  Value=0
  WindZ : Constant  Value=0
  XY Graph : Record  NumPorts=2.0  FileSettingsInternal="{\"entries\":[{\"content\":{\"excelSettings\":{\"content\":{},\"type\":\"Streamout.ExcelSettings\"},\"parquetSettings\":{\"content\":{},\"type\":\"Streamout.ParquetSettings\"}},\"type\":\"Streamout.FileSettingStorage\",\"uuid\":\"\"}],\"packageUris\":[\"http:\\/\\/schema.mathworks.com\\/mf0\\/streamout_blocks\\/R2020a\"],\"version\":\"1.0\"}"  FrameSettings=[0, 0]  Layout=[1 1]  SignalsInternal="{\"entries\":[{\"content\":{\"signals\":[{\"content\":{\"blockPath\":[],\"dimensions\":[1],\"domain\":\"\",\"lineColor\":\"#a2142f\",\"plots\":[ 1 ],\"port\":1,\"sid\":[\"\"],\"signalID\":1,\"signalName\":\"<Y>\"},\"type\":\"RecordBlkView.Signal\",\"uuid\":\"\"},{\"content\":{\"blockPath\":[],\"dimensions\":[1],\"domain\":\"\",\"lineColor\":\"#139fff\",\"plots\":[ 1 ],\"port\":2,\"sid\":[\"\"],\"signalID\":2,\"signalName\":\"<X>\"},\"type\":\"RecordBlkView.Signal\",\"uuid\":\"\"}]},\"type\":\"RecordBlkView.InputSignals\",\"uuid\":\"\"}],\"packageUris\":[\"http:\\/\\/schema.mathworks.com\\/mf0\\/streamout_blocks\\/R2020a\"],\"version\":\"1.0\"}"  VisualizationBindings="{\"xyplotplugin\":{\"info\":[{\"series\":[{\"bindingParametersList\":[{\"parameter\":\"X-Axis\",\"signalID\":1,\"signalName\":\"<Y>\"},{\"parameter\":\"Y-Axis\",\"signalID\":2,\"signalName\":\"<X>\"}],\"seriesID\":0}],\"subplotID\":1}]}}"  CompatibilityTag=XY
  axles_dist : Constant  Value=EV.RearAxlePositionfromCG + EV.FrontAxlePositionfromCG
  fi : Constant
  g : Constant  Value=9.81
  on/off : ManualSwitch
  on/off1 : ManualSwitch  CurrentSetting=0
  on/off2 : ManualSwitch  CurrentSetting=0
  radius : Constant  Value=WHL.LoadedRadius
  wires:
  WindX/1 -> Bus Creator/1
  WindZ/1 -> Bus Creator/3
  WindY/1 -> Bus Creator/2
  Bus Creator/1 -> [Wind]
  [Wind] -> Vehicle Body 3DOF Dual Track/4
  MATLAB Function/1(y) -> [Friction]
  [Friction] -> Vehicle Body 3DOF Dual Track/5
  GND.Friction/1 -> MATLAB Function/1(u)
  Constant3/1 -> Mapped Motor (Left)/1
  Constant1/1 -> Mapped Motor (Right)/1
  Constant/1 -> [omega_RLwheel]
  [xdot] -> Relação de Transmissão_/1
  [xdot] -> Relação de Transmissão/1
  Constant2/1 -> [omega_RRwheel]
  Constant13/1 -> [FL_Speed]
  Constant14/1 -> [FR_Speed]
  [Atrito_L] -> Min1/1
  [Atrito_R] -> Min1/2
  [Atrito] -> Scope/1  "Atrito"
  From11/1 -> Sum of Elements6/1
  From12/1 -> Sum of Elements6/2
  Sum of Elements6/1 -> Gain6/1
  Gain6/1 -> Goto11/1
  ./1 -> [steering_angle]
  [desired_yaw] -> Scope1/1  "desired_yaw"
  [max_yaw] -> Scope2/1  "max_yaw"
  [SR_L] -> Scope3/1  "SR_L"
  [SR_R] -> Scope3/2  "SR_R"
  [Atrito_L] -> Scope4/1  "Atrito_L"
  [Atrito_R] -> Scope5/1  "Atrito_R"
  MATLAB Function8/1(VT_Setpoint) -> Scope19/1, [VT_setpoint]
  Abs/1 -> Switch2/3
  on/off/1 -> Abs/1, Switch2/2, Abs1/1, Switch1/2
  Abs1/1 -> Switch1/1
  Saturation3/1 -> Manual Switch3/1
  Saturation2/1 -> Manual Switch4/1
  [VT_Error] -> PID Controller1/1
  Ground6/1 -> on/off/2
  Switch2/1 -> Saturation2/1, Manual Switch4/2
  Ground4/1 -> Switch1/3, Switch2/1
  Manual Switch3/1 -> [RightTrq_VT]
  Manual Switch4/1 -> [LeftTrq_VT]
  Switch1/1 -> Saturation3/1, Manual Switch3/2  "RightTorqueVT"
  PID Controller1/1 -> Scope17/1, on/off/1
  [FR_Speed] -> MATLAB Function1/2(FR_speed)
  [FL_Speed] -> MATLAB Function1/1(FL_speed)
  [omega_RLwheel] -> MATLAB Function1/3(omega_RLwheel)
  [omega_RRwheel] -> MATLAB Function1/4(omega_RRwheel)
  radius/1 -> MATLAB Function1/5(radius)
  MATLAB Function1/2(SR_R) -> [SR_R]
  MATLAB Function1/1(SR_L) -> [SR_L]
  Constant4/1 -> MATLAB Function2/2(C1)
  Constant16/1 -> MATLAB Function2/3(C2)
  Constant17/1 -> MATLAB Function2/4(C3)
  [SR_L] -> MATLAB Function2/1(SR_L)
  MATLAB Function2/1(Atrito_L) -> [Atrito_L]
  MATLAB Function3/1(Atrito_R) -> [Atrito_R]
  Constant19/1 -> MATLAB Function3/4(C3)
  Constant18/1 -> MATLAB Function3/3(C2)
  Constant20/1 -> MATLAB Function3/2(C1)
  [SR_R] -> MATLAB Function3/1(SR_R)
  [AvgSteer] -> MATLAB Function4/1(steering_angle)
  [Vcg] -> MATLAB Function4/2(Vcg)
  Ku/1 -> MATLAB Function4/3(Ku)
  axles_dist/1 -> MATLAB Function4/4(axles_dist)
  MATLAB Function4/1(desired_yaw) -> [desired_yaw]
  g/1 -> MATLAB Function5/4(g)
  [Vcg] -> MATLAB Function5/3(Vcg)
  fi/1 -> MATLAB Function5/5(fi)
  MATLAB Function5/1(max_yaw) -> [max_yaw]
  [Atrito] -> MATLAB Function5/2(atrito)
  Vehicle Body 3DOF Dual Track/5 -> [real_YawRate]
  [VT_setpoint] -> Subtract/1
  [real_YawRate] -> Subtract/2
  Subtract/1 -> Scope20/1, [VT_Error]
  [LeftTrq_VT] -> Scope6/1  "LeftTorqueVT"
  [RightTrq_VT] -> Scope6/2  "RightTorqueVT"
  Mapped Motor (Left)/1 -> Terminator/1
  Mapped Motor (Right)/1 -> Terminator1/1
  Mapped Motor (Right)/3 -> Gain/1
  Mapped Motor (Left)/3 -> Gain1/1
  Mapped Motor (Right)/2 -> Terminator2/1
  Mapped Motor (Left)/2 -> Terminator3/1
  Engine Response1/1 -> Scope11/2, [RightMtrTrq]  "RightMtrTrq"
  Engine Response2/1 -> Scope11/1, [LeftMtrTrq]  "LeftMtrTrq"
  Vector Concatenate/1 -> Vehicle Body 3DOF Dual Track/3
  Constant5/1 -> Vector Concatenate1/1, Vector Concatenate1/2
  Vector Concatenate1/1 -> Vehicle Body 3DOF Dual Track/2
  Vehicle Body 3DOF Dual Track/3 -> [ydot]
  Vehicle Body 3DOF Dual Track/6 -> Terminator8/1
  Vehicle Body 3DOF Dual Track/7 -> Terminator9/1
  Constant7/1 -> Scope15/1, Sum/1
  [RightTrq_VT] -> Scope15/2, Sum/2
  [LeftTrq_VT] -> Scope14/2, Sum1/2
  Signal Specification8/1 -> Scope7/2, Vector Concatenate2/2, Sum of Elements/1  "right_angle"
  MATLAB Function6/1(left_wheel_angle) -> Signal Specification7/1
  Signal Specification7/1 -> Sum of Elements/2, Vector Concatenate2/1, Scope7/1  "lef_angle"
  MATLAB Function6/2(right_wheel_angle) -> Signal Specification8/1
  Saturation/1 -> Scope14/4, Mapped Motor (Left)/3  "TrqCmdL"
  Sum/1 -> Scope15/3, Saturation1/1
  Constant6/1 -> Scope14/1, Sum1/1
  Sum1/1 -> Scope14/3, Saturation/1
  [steering_angle] -> MATLAB Function6/1(steering_angle)
  Vehicle Body 3DOF Dual Track/1 -> [Chassi_info]
  [Chassi_info] -> 2D Visualization/1(Inport)
  Vehicle Body 3DOF Dual Track/2 -> [xdot]
  Vehicle Body 3DOF Dual Track/4 -> [psi]
  Vector Concatenate2/1 -> [WhlAngF]
  [WhlAngF] -> Vehicle Body 3DOF Dual Track/1
  Subtract1/1 -> [CA_error_left]
  CA_setpoint/1 -> Subtract1/1
  [SR_L] -> Subtract1/2
  Subtract2/1 -> [CA_error_right]
  CA_setpoint1/1 -> Subtract2/1
  [SR_R] -> Subtract2/2
  [CA_error_left] -> Scope12/1
  [CA_error_right] -> Scope12/2
  [CA_error_left] -> PID Controller2/1
  [CA_error_right] -> PID Controller3/1
  Ground1/1 -> on/off1/2
  PID Controller3/1 -> on/off1/1
  Ground2/1 -> on/off2/2
  PID Controller2/1 -> on/off2/1
  Sum of Elements/1 -> Gain4/1
  Gain4/1 -> [AvgSteer]
  Signal Specification4/1 -> Mapped Motor (Right)/2
  Relação de Transmissão/1 -> Signal Specification4/1
  Relação de Transmissão_/1 -> Signal Specification1/1
  Signal Specification1/1 -> Mapped Motor (Left)/2
  [xdot] -> MATLAB Function7/1(xdot)
  [ydot] -> MATLAB Function7/2(ydot)
  [psi] -> Scope21/1, MATLAB Function7/3(psi)
  [xdot] -> Scope13/1, [Vcg]
  Integrator1/1 -> Vehicle Position/1
  Integrator4/1 -> Vehicle Position/2
  MATLAB Function7/1(Vx) -> Scope10/2, Integrator1/1  "SpeedYaxle"
  MATLAB Function7/2(Vy) -> Scope10/1, Integrator4/1  "SpeedXaxle"
  Gain/1 -> Engine Response1/1
  Gain1/1 -> Engine Response2/1
  [real_YawRate] -> Scope9/1  "real_yaw_rate"
  [VT_setpoint] -> Scope9/2  "Setpoint"
  Saturation1/1 -> Mapped Motor (Right)/3, Scope15/4  "TrqCmdR"
  Abs3/1 -> Switch3/1
  Ground3/1 -> Switch3/3
  on/off2/1 -> Scope8/1, Abs3/1, Switch3/2
  Abs2/1 -> Switch4/1
  Ground5/1 -> Switch4/3
  on/off1/1 -> Scope8/2, Abs2/1, Switch4/2
  Switch3/1 -> [LeftTrq_CA]
  Switch4/1 -> [RightTrq_CA]
  [LeftTrq_CA] -> Scope16/1  "LeftTrq_CA"
  [RightTrq_CA] -> Scope16/2  "RightTrq_CA"
  Manual Switch/1 -> [Atrito]
  Min1/1 -> Manual Switch/2
  Constant8/1 -> Manual Switch/1
  [LeftMtrTrq] -> Vector Concatenate/1
  [RightMtrTrq] -> Vector Concatenate/2
  [LeftMtrTrq] -> Scope18/1  "Trq_Left"
  [RightMtrTrq] -> Scope18/2  "Trq_Right"
  [steering_angle] -> MATLAB Function5/1(angle)
  [desired_yaw] -> MATLAB Function8/1(desired_yaw)
  [max_yaw] -> MATLAB Function8/2(max_yaw)
  Bus Selector/2 -> XY Graph/2  "<X>"
  [Chassi_info] -> Bus Selector/1
  Bus Selector/1 -> XY Graph/1  "<Y>"

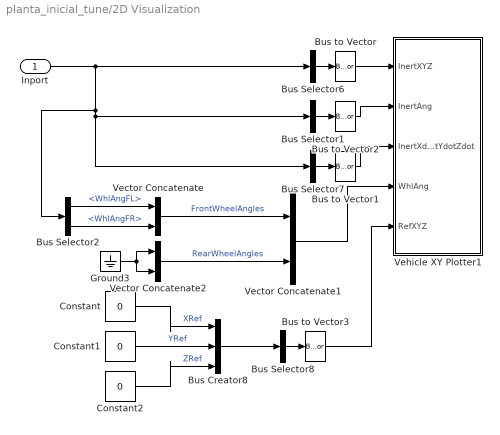
== system planta_inicial_tune/2D Visualization ==
  Inport : Inport
  Bus Creator8 : BusCreator  Inputs=3
  Bus Selector1 : BusSelector  OutputSignals=InertFrm.Cg.Ang.phi,InertFrm.Cg.Ang.theta,InertFrm.Cg.Ang.psi  OutputAsBus=on
  Bus Selector2 : BusSelector  OutputSignals=BdyFrm.FrntAxl.Steer.WhlAngFL,BdyFrm.FrntAxl.Steer.WhlAngFR
  Bus Selector6 : BusSelector  OutputSignals=InertFrm.Geom.Disp.X,InertFrm.Geom.Disp.Y,InertFrm.Geom.Disp.Z  OutputAsBus=on
  Bus Selector7 : BusSelector  OutputSignals=InertFrm.Geom.Vel.Xdot,InertFrm.Geom.Vel.Ydot,InertFrm.Geom.Vel.Zdot  OutputAsBus=on
  Bus Selector8 : BusSelector  OutputSignals=XRef,YRef,ZRef  OutputAsBus=on
  Bus to Vector{,1..3} (4 alike) : BusToVector
  Constant : Constant  Value=0
  Constant1 : Constant  Value=0
  Constant2 : Constant  Value=0
  Ground3 : Ground
  Vector Concatenate : Concatenate
  Vector Concatenate1 : Concatenate
  Vector Concatenate2 : Concatenate
  Vehicle XY Plotter1 : Subsystem  mask(Vehicle XY Plotter){extRef=on, extStats=off, extTireF=off, a=EV.FrontAxlePositionfromCG, b=EV.RearAxlePositionfromCG, w=1.17, figBorder=10, bufferSize=1024, velNorm=5, tireFNorm=1000, pltDT=0.1}
      mask prompts: extRef "Plot path reference, extRef"; extStats "Display speed, RPM and Gear"; extTireF "Display tire forces"; a "Distance to front axle from CG, a [m]:"; b "Distance to rear axle from CG, b [m]:"; w "Track width, w [m]:"; figBorder "Distance to figure borders, figBorder [m]:"; bufferSize "Path buffer sampe size, bufferSize []:"; velNorm "Velocity vector scaling, velNorm [m*s/m]:"; tireFNorm "Tire force vector scaling, tireFNorm [m/N]:"; pltDT "Plot update rate, pltDT [s]:"
      mask help:
      | This block will display a MATLAB figure which indicates the vehicle path, current position and heading velocity.
      | An optional path reference is also provided.
      mask init:
      | block = gcb;
      | if autoblkschecksimstopped(block)
      |     ParamNames = {'extRef';'extStats';'extTireF';'extTireF'};
      |     PortNames = {'RefXYZ';'Stats';'TireFx';'TireFy'};
      |     for idx=1:length(PortNames)
      |         InportOption  = {'built-in/Ground', [PortNames{idx}, ' Ground'];...
      |             'built-in/Inport',PortNames{idx}};
      |         if ~strcmp(get_param(block,ParamNames{idx}),'on')
      |             NewBlkHdl = autoblksreplaceblock(block, InportOption, 1);
      |             set_param(NewBlkHdl, 'ShowName', 'off');
      |         else
      |             autoblksreplaceblock(block, InportOption, 2);
      |         end
      |     end
      |     InportNames = {'InertXYZ';'InertAng';'InertXdotYdotZdot';'WhlAng';'RefXYZ';'Stats';'TireFx';'TireFy'};
      |     FoundNames = get_param(find_system(block, 'LookUnderMasks', 'all', 'SearchDepth', 1, 'FollowLinks', 'on', 'BlockType', 'Inport'), 'Name');
      |     [~,PortI] = intersect(InportNames, FoundNames);
      |     PortI = sort(PortI);
      |     for idx = 1:length(PortI)
      |         set_param([block, '/', InportNames{PortI(idx)}], 'Port', num2str(idx));
      |     end
      | end
      mask TypeOptions a: Vehicle XY Plotter/a
      mask TypeOptions b: Vehicle XY Plotter/b
      mask TypeOptions w: Vehicle XY Plotter/w
      mask TypeOptions figBorder: Vehicle XY Plotter/figBorder
      mask TypeOptions bufferSize: Vehicle XY Plotter/bufferSize
      mask TypeOptions velNorm: Vehicle XY Plotter/velNorm
      mask TypeOptions tireFNorm: Vehicle XY Plotter/tireFNorm
      mask DialogControl Container3 Prompt: Plot and Display Options
  wires:
  Vector Concatenate1/1 -> Vehicle XY Plotter1/4(WhlAng)
  Ground3/1 -> Vector Concatenate2/1, Vector Concatenate2/2
  Bus Selector6/1 -> Bus to Vector/1
  Vector Concatenate/1 -> Vector Concatenate1/1  "FrontWheelAngles"
  Vector Concatenate2/1 -> Vector Concatenate1/2  "RearWheelAngles"
  Bus Selector7/1 -> Bus to Vector1/1
  Bus to Vector1/1 -> Vehicle XY Plotter1/3(InertXdotYdotZdot)
  Bus to Vector/1 -> Vehicle XY Plotter1/1(InertXYZ)
  Bus to Vector2/1 -> Vehicle XY Plotter1/2(InertAng)
  Bus Selector1/1 -> Bus to Vector2/1
  Inport/1 -> Bus Selector2/1, Bus Selector7/1, Bus Selector1/1, Bus Selector6/1
  Bus Selector2/1 -> Vector Concatenate/1  "<WhlAngFL>"
  Bus Selector2/2 -> Vector Concatenate/2  "<WhlAngFR>"
  Bus Creator8/1 -> Bus Selector8/1
  Bus Selector8/1 -> Bus to Vector3/1
  Constant2/1 -> Bus Creator8/3  "ZRef"
  Constant1/1 -> Bus Creator8/2  "YRef"
  Bus to Vector3/1 -> Vehicle XY Plotter1/5(RefXYZ)
  Constant/1 -> Bus Creator8/1  "XRef"

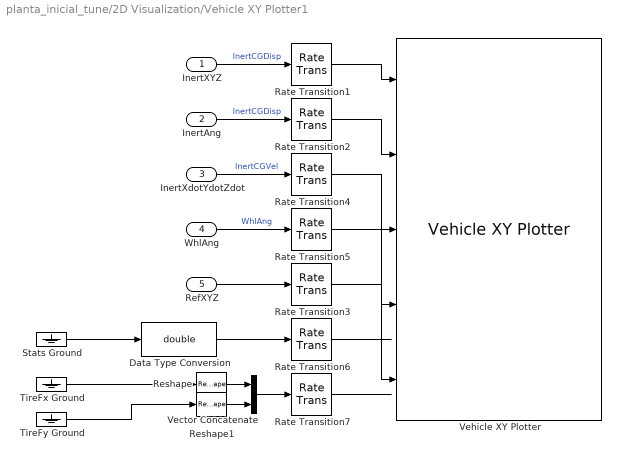
== system planta_inicial_tune/2D Visualization/Vehicle XY Plotter1 ==
  InertXYZ : Inport
  InertAng : Inport  Port=2
  InertXdotYdotZdot : Inport  Port=3
  WhlAng : Inport  Port=4
  RefXYZ : Inport  Port=5
  Data Type Conversion : DataTypeConversion  OutDataTypeStr=double  SaturateOnIntegerOverflow=off  RndMeth=Floor
  Rate Transition{1..7} (7 alike) : RateTransition  Deterministic=off  OutPortSampleTime=pltDT
  Reshape : Reshape  OutputDimensionality=Row vector (2-D)
  Reshape1 : Reshape  OutputDimensionality=Row vector (2-D)
  Stats Ground : Ground
  TireFx Ground : Ground
  TireFy Ground : Ground
  Vector Concatenate : Concatenate  Mode=Multidimensional array
  Vehicle XY Plotter : vehdynlibviscommon/Vehicle XY Plotter  w=w  a=a  b=b  figBorder=figBorder  bufferSize=bufferSize  extStats=off  extTireF=off
  wires:
  Vector Concatenate/1 -> Rate Transition7/1
  Reshape1/1 -> Vector Concatenate/2
  Reshape/1 -> Vector Concatenate/1
  RefXYZ/1 -> Rate Transition3/1
  Rate Transition7/1 -> ?
  Data Type Conversion/1 -> Rate Transition6/1
  Rate Transition6/1 -> ?
  Rate Transition5/1 -> Vehicle XY Plotter/4
  Rate Transition4/1 -> Vehicle XY Plotter/3
  Rate Transition2/1 -> Vehicle XY Plotter/2
  Rate Transition1/1 -> Vehicle XY Plotter/1
  Rate Transition3/1 -> Vehicle XY Plotter/5
  WhlAng/1 -> Rate Transition5/1  "WhlAng"
  InertXYZ/1 -> Rate Transition1/1  "InertCGDisp"
  InertXdotYdotZdot/1 -> Rate Transition4/1  "InertCGVel"
  InertAng/1 -> Rate Transition2/1  "InertCGDisp"
  Stats Ground/1 -> Data Type Conversion/1
  TireFx Ground/1 -> Reshape/1
  TireFy Ground/1 -> Reshape1/1

== matlab function planta_inicial_tune/MATLAB Function1 ==
  data: FL_speed input; FR_speed input; SR_L output; omega_RLwheel input; omega_RRwheel input; radius input; SR_R output
function [SR_L , SR_R] = fcn(FL_speed, FR_speed, omega_RLwheel, omega_RRwheel, radius)

SR_L = (omega_RLwheel * radius/FL_speed)-1;
SR_R = (omega_RRwheel * radius/FR_speed)-1;

== matlab function planta_inicial_tune/MATLAB Function ==
  data: u input; y output
function y = fcn(u)

y = [u(1), u(2); u(3), u(4)];

== matlab function planta_inicial_tune/MATLAB Function2 ==
  data: SR_L input; Atrito_L output; C1 input; C2 input; C3 input
function Atrito_L = fcn(SR_L, C1, C2, C3)

Atrito_L = (C1*(1-(exp(SR_L*C2*(-1)))))-(C3*SR_L);

== matlab function planta_inicial_tune/MATLAB Function3 ==
  data: SR_R input; Atrito_R output; C1 input; C2 input; C3 input
function Atrito_R = fcn(SR_R, C1, C2, C3)

Atrito_R = (C1*(1-(exp(SR_R*C2*(-1)))))-(C3*SR_R);

== matlab function planta_inicial_tune/MATLAB Function4 ==
  data: steering_angle input; desired_yaw output; Vcg input; Ku input; axles_dist input
function desired_yaw = fcn(steering_angle, Vcg, Ku, axles_dist)

desired_yaw = (Vcg*steering_angle)/(axles_dist+(Ku*Vcg*Vcg));

== matlab function planta_inicial_tune/MATLAB Function5 ==
  data: angle input; atrito input; max_yaw output; Vcg input; g input; fi input
function max_yaw = fcn(angle, atrito, Vcg, g, fi)

if angle >= 0
    a = 1;
else
    a = -1;
end

max_yaw = a*(fi*atrito*g)/(Vcg);

== matlab function planta_inicial_tune/MATLAB Function6 ==
  data: left_wheel_angle output; steering_angle input; right_wheel_angle output
function [left_wheel_angle, right_wheel_angle] = fcn(steering_angle)

if(steering_angle<=0)
    left_wheel_angle = 0.30732918494924799*steering_angle;
    right_wheel_angle = 0.268948751217872*steering_angle;

else (steering_angle>0)
    left_wheel_angle = 0.268948678266664*steering_angle;
    right_wheel_angle = 0.30732915888671*steering_angle;
end
end

== matlab function planta_inicial_tune/MATLAB Function7 ==
  data: xdot input; Vx output; ydot input; Vy output; psi input
function [Vx, Vy] = fcn(xdot, ydot, psi)

Vx = (xdot*cos(psi)) + (ydot*sin(psi));
Vy = (xdot*sin(psi)) + (ydot*cos(psi));

== matlab function planta_inicial_tune/MATLAB Function8 ==
  data: desired_yaw input; max_yaw input; VT_Setpoint output
function VT_Setpoint = fcn(desired_yaw, max_yaw)

if desired_yaw >= 0
    VT_Setpoint = min(desired_yaw, max_yaw);
else
    VT_Setpoint = max(desired_yaw, max_yaw);
end
